simulink model "AMR_ID_BoucWen"  (R2021a)
settings: Solver=ode8  StartTime=0.0  StopTime=totaltime  FixedStep=dtsim  RelTol=1e-3
model workspace (MAT data in the model file):
  unnamed = 0
values from neighbouring files (symbols this model uses):
  i = Data.Amp    [MR_BoucWen.m]
undefined symbols (not defined in the file or in its folder): params
settings Model: PauseTimes=8  OrderedModelArguments=off  Creator=cristobal  LastModifiedBy=maryf
settings SolverCC: NumberNewtonIterations=40  ConcurrentTasks=on  AlgebraicLoopSolver=TrustRegion  PositivePriorityOrder=on
settings DataIOCC: ReturnWorkspaceOutputs=off
settings OptimizationCC: BlockReduction=off  OptimizeBlockIOStorage=off
settings DebuggingCC: IgnoredZcDiagnostic=none  SFMachineParentedDataDiag=warning  ArithmeticOperatorsInVariantConditions=warning
settings HardwareCC: ProdBitPerLong=64  ProdLongLongMode=on  ProdHWDeviceType=Intel->x86-64 (Linux 64)
settings SFSimCC: SimUseLocalCustomCode=off  CustomCodeUndefinedFunction=UseInterfaceOnly
settings RTWCC: Description=Simulink Real-Time  SystemTargetFile=slrealtime.tlc  TemplateMakefile=slrealtime_default_tmf  RTWUseLocalCustomCode=off  Toolchain=Simulink Real-Time Toolchain  BuildConfiguration=Faster Runs  CodeExecutionProfiling=on  TargetLang=C++
settings CodeAppCC: StateflowObjectComments=on

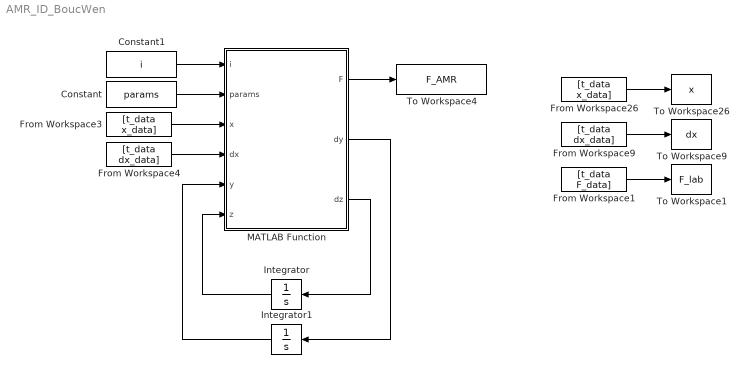
== system AMR_ID_BoucWen ==
  Constant : Constant  Value=params
  Constant1 : Constant  Value=i
  From Workspace1 : FromWorkspace  VariableName=[t_data F_data]
  From Workspace26 : FromWorkspace  VariableName=[t_data x_data]
  From Workspace3 : FromWorkspace  VariableName=[t_data x_data]
  From Workspace4 : FromWorkspace  VariableName=[t_data dx_data]
  From Workspace9 : FromWorkspace  VariableName=[t_data dx_data]
  Integrator : Integrator
  Integrator1 : Integrator
  MATLAB Function : MATLAB Function  TreatAsAtomicUnit=on
  To Workspace1 : ToWorkspace  VariableName=F_lab  SaveFormat=Timeseries  SampleTime=-1
  To Workspace26 : ToWorkspace  VariableName=x  SaveFormat=Timeseries  SampleTime=-1
  To Workspace4 : ToWorkspace  VariableName=F_AMR  SaveFormat=Timeseries  SampleTime=-1
  To Workspace9 : ToWorkspace  VariableName=dx  SaveFormat=Timeseries  SampleTime=-1
  wires:
  From Workspace9/1 -> To Workspace9/1
  From Workspace26/1 -> To Workspace26/1
  From Workspace4/1 -> MATLAB Function/4(dx)
  From Workspace3/1 -> MATLAB Function/3(x)
  From Workspace1/1 -> To Workspace1/1
  MATLAB Function/1(F) -> To Workspace4/1
  MATLAB Function/3(dz) -> Integrator/1
  MATLAB Function/2(dy) -> Integrator1/1
  Integrator/1 -> MATLAB Function/6(z)
  Integrator1/1 -> MATLAB Function/5(y)
  Constant/1 -> MATLAB Function/2(params)
  Constant1/1 -> MATLAB Function/1(i)

== matlab function AMR_ID_BoucWen/MATLAB Function ==
  data: i input; params input; x input; dx input; y input; z input; F output size=1; dy output; dz output
function [F,dy,dz] = fcn(i,params,x,dx,y,z)
    A        = 300;   
    k0       = 0;               %N/mm
    k1       = 0;               %N/mm
    x0       = 0;               %mm
    n        = 2;   
    alpha    = params(1);       %N/mm
    beta     = params(2);       %mm^-2
    gamma    = beta;            %mm^-2
    c0       = params(3);       %Ns/mm
    c1       = params(4);       %Ns/mm


    dy = 1/(c0+c1)*(alpha*z+k0*(x-y)+c0*dx);
    dz = -gamma*abs(dx-dy)*((abs(z))^(n-1))*z-beta*(dx-dy)*(abs(z)^n)+A*(dx-dy);
    F  = c1*dy+k1*(x-x0);
